simulink model "Symmetry_Inverter"  (Simulink 8.3)
settings: Solver=ode23tb  StartTime=0.0  StopTime=tfin  RelTol=1e-4
values from neighbouring files (symbols this model uses):
  amp_feedback_saturation = 400    [Symmetry_ini_COPY.m]
  Butterworth_filter_order = 8    [Sketch_controller_model_ini.m]    (also in Symmetry_ini.m; Symmetry_ini_COPY.m)
  C_Network = [0, 0, 0]    [Symmetry_ini.m]    (also in Symmetry_ini_COPY.m)
  Capacitive_Load_R_RC = [30e-3,  60e-3,  40e-3;                                1e-3, 5e-3, 3e-3]    [Symmetry_ini.m]    (also in Symmetry_ini_COPY.m = [60e-3,  120e-3,  80e-3;                                 1e-)
  Capacitive_Load_S_RC = [30e-3,  60e-3,  40e-3;                                1e-3, 5e-3, 3e-3]    [Symmetry_ini.m]    (also in Symmetry_ini_COPY.m = [60e-3,  120e-3,  80e-3;                                1e-3)
  Capacitive_Load_T_RC = [30e-3,  60e-3,  40e-3;                                1e-3, 5e-3, 3e-3]    [Symmetry_ini.m]    (also in Symmetry_ini_COPY.m = [60e-3,  120e-3,  80e-3;                                 1e-)
  i = str2num(answer{1})/sample    [Test_intersect.m]
  initial_value = [0.00,0.00,0.00,                  0,0,0]    [Symmetry_ini_COPY.m]
  L_Network = [3.185e-3, 3.185e-3, 3.185e-3, 3.185e-3]    [Symmetry_ini.m]    (also in Symmetry_ini_COPY.m)
  L_Source = [3.185e-3, 3.185e-3, 3.185e-3]    [Sketch_controller_model_ini.m]    (also in Symmetry_ini.m; Symmetry_ini_COPY.m)
  Load_R = [50,50,50]    [Symmetry_ini.m]    (also in Symmetry_ini_COPY.m)
  Load_RL = [35.35,   35.35,   35.35;                  0.1125,  0.1125,  0.1125]    [Symmetry_ini.m]    (also in Symmetry_ini_COPY.m = [35.35,   35.35,   35.35;                   0.1125,  0.1125,)
  Load_Wire_Resistance = [0.1,0.2]    [Symmetry_ini.m]    (also in Symmetry_ini_COPY.m)
  P_gain = 0.00001    (= 1e-05)    [Symmetry_ini_COPY.m]
  phase_feedback_saturation = pi    (= 3.14159265359)    [Symmetry_ini_COPY.m]
  Phase_Source = [0,2/3*pi,4/3*pi]    [Sketch_controller_model_ini.m]    (also in Symmetry_REAL_TIME_ini.m = [0,-2/3*pi,-4/3*pi]; Symmetry_ini.m; Symmetry_ini_COPY.m = [0,-2/3*pi,-4/3*pi])
  PowerGain = 2e-3    (= 0.002)    [Symmetry_ini_COPY.m]
  PowerGain_UpperLimit = 10    [Symmetry_ini_COPY.m]
  R_Network = [0.4, 0.4, 0.4, 0.4]    [Symmetry_ini.m]    (also in Symmetry_ini_COPY.m)
  R_Source = [0.4, 0.4, 0.4]    [Sketch_controller_model_ini.m]    (also in Symmetry_ini.m; Symmetry_ini_COPY.m)
  sample = 10e-5    (= 0.0001)    [Inverter_ini.m]    (also in Sketch_controller_model_ini.m; Symmetry_REAL_TIME_ini.m; Symmetry_ini.m; Symmetry_ini_COPY.m)
  Source_Frequency = [50,50,50]    [Sketch_controller_model_ini.m]    (also in Symmetry_ini.m; Symmetry_ini_COPY.m)
  Start_Control = 1    [Symmetry_ini_COPY.m]
  START_Load_R = [0.001,100,100]    [Symmetry_ini_COPY.m]
  START_Load_RC = [100,100,0.001]    [Symmetry_ini_COPY.m]
  START_Load_RL = [100,0.001,100]    [Symmetry_ini_COPY.m]
  step_size = [5,5,5,                  0.36,0.36,0.36]    [Symmetry_ini_COPY.m]
  test_step = [0.5,0.5,0.5,                  0.02,0.02,0.02]    [Symmetry_ini_COPY.m]
  U_PV_MAX = 600    [Symmetry_ini_COPY.m]
  Urms_Source = [230,230,230]    [Sketch_controller_model_ini.m]    (also in Symmetry_REAL_TIME_ini.m; Symmetry_ini.m; Symmetry_ini_COPY.m)
libraries: powerlib x95, simulink x18, powerlib_extras x12, dspsigops x10, commsequence2 x6, dsparch4 x4, dspxfrm3 x3, powerlib_meascontrol x2
(part 1 of 2)
settings Model: Creator=gorbep  LastModifiedBy=Templomos  SimulationMode=accelerator
settings SolverCC: SolverResetMethod=Robust
settings DataIOCC: SignalLoggingSaveFormat=Dataset
settings OptimizationCC: SimCompilerOptimization=On
settings DebuggingCC: UnderspecifiedInitializationDetection=Simplified  StateNameClashWarn=none
settings GRTTargetCC: CombineOutputUpdateFcns=on  GRTInterface=off

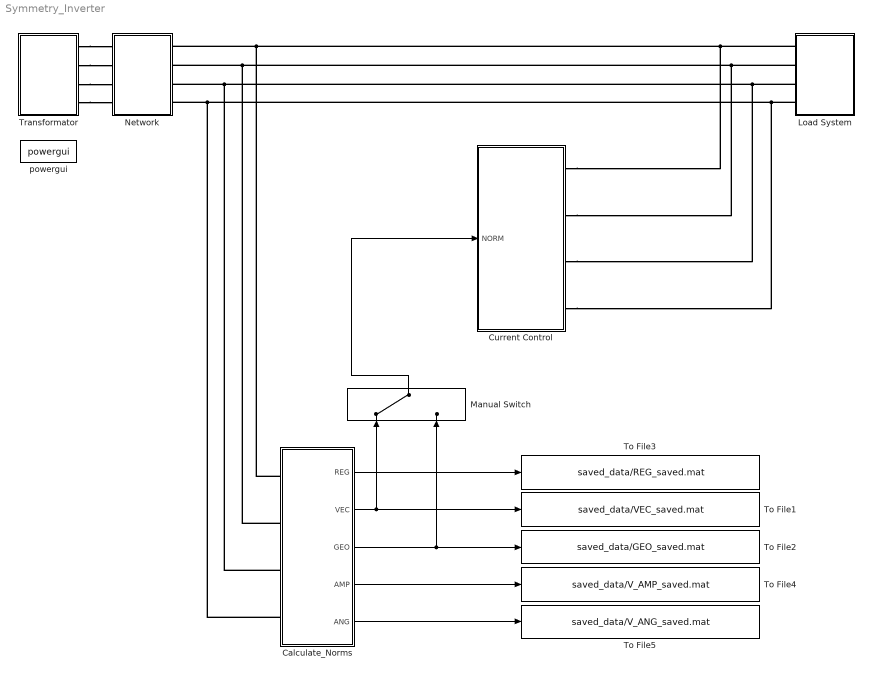
== system Symmetry_Inverter ==
  Calculate_Norms : Subsystem
  Current Control : Subsystem
  Load System : Subsystem
  Manual Switch : ManualSwitch
  Network : Subsystem
  To File1 : ToFile  Filename=saved_data/VEC_saved.mat  MatrixName=VEC_saved  SaveFormat=Timeseries  SampleTime=sample
  To File2 : ToFile  Filename=saved_data/GEO_saved.mat  MatrixName=GEO_saved  SaveFormat=Timeseries  SampleTime=sample
  To File3 : ToFile  Filename=saved_data/REG_saved.mat  MatrixName=REG_saved  SaveFormat=Timeseries  SampleTime=sample
  To File4 : ToFile  Filename=saved_data/V_AMP_saved.mat  MatrixName=V_AMP_saved  SaveFormat=Timeseries  SampleTime=sample
  To File5 : ToFile  Filename=saved_data/V_ANG_saved.mat  MatrixName=V_ANG_saved  SaveFormat=Timeseries  SampleTime=sample
  Transformator : Subsystem
  powergui : powerlib/powergui  SimulationMode=Continuous  SolverType=Tustin  SampleTime=50e-6  frequency=60  SPID=off  DisableSnubberDevices=off  DisableRonSwitches=off  DisableVfSwitches=off  SwTol=0  Interpol=off  DisplayEquations=off  Ts=0  methode=off  frequencyindice=0  Pbase=100e6  ErrMax=1e-4  Iterations=50  UnitsV=kV  UnitsW=MW  FunctionMessages=off  echomessages=off  HookPort=off  EnableUseOfTLC=off  x0status=blocks  RestoreLinks=warning  ResistiveCurrentMeasurement=off  Frange=[0:2:500]  Ylog=off  Xlog=on  ShowGrid=off  save=off  variable=ZData  structure=0  ZoomFFT=on  StartTime=0.0  cycles=1  DisplayStyle=1  fundamental=60  FreqAxis=off  MaxFrequency=1000  frequencyindicesteady=1  RmsSteady=1  display=off
  wires:
  Calculate_Norms/1(REG) -> To File3/1
  Calculate_Norms/3(GEO) -> Manual Switch/2, To File2/1
  Calculate_Norms/2(VEC) -> Manual Switch/1, To File1/1
  Calculate_Norms/4(AMP) -> To File4/1
  Calculate_Norms/5(ANG) -> To File5/1
  Manual Switch/1 -> Current Control/1(NORM)
  connections:
  Transformator/RConn1 -- Network/LConn1
  Transformator/RConn2 -- Network/LConn2
  Transformator/RConn3 -- Network/LConn3
  Transformator/RConn4 -- Network/LConn4
  Load System/LConn1 -- Calculate_Norms/LConn1 -- Network/RConn1 -- Current Control/RConn1
  Load System/LConn2 -- Calculate_Norms/LConn2 -- Network/RConn2 -- Current Control/RConn2
  Load System/LConn3 -- Calculate_Norms/LConn3 -- Network/RConn3 -- Current Control/RConn3
  Load System/LConn4 -- Network/RConn4 -- Calculate_Norms/LConn4 -- Current Control/RConn4

== system Symmetry_Inverter/Calculate_Norms ==
  Mearusement_calc : Subsystem
  Sources1 : ToWorkspace  VariableName=V_conn  SaveFormat=Structure With Time  SampleTime=sample
  Voltage Measurement : powerlib/Measurements/Voltage Measurement  PhasorSimulation=off  OutputType=Complex  PSBequivalent=0
  Voltage Measurement1 : powerlib/Measurements/Voltage Measurement  PhasorSimulation=off  OutputType=Complex  PSBequivalent=0
  Voltage Measurement2 : powerlib/Measurements/Voltage Measurement  PhasorSimulation=off  OutputType=Complex  PSBequivalent=0
  R : PMIOPort  Port=1  Side=Left
  S : PMIOPort  Port=2  Side=Left
  T : PMIOPort  Port=3  Side=Left
  N : PMIOPort  Port=4  Side=Left
  REG : Outport
  VEC : Outport  Port=2
  GEO : Outport  Port=3
  AMP : Outport  Port=4
  ANG : Outport  Port=5
  wires:
  Voltage Measurement/1 -> Mearusement_calc/1(V_R)
  Voltage Measurement1/1 -> Mearusement_calc/2(V_S)
  Voltage Measurement2/1 -> Mearusement_calc/3(V_T)
  Mearusement_calc/1(Voltage) -> Sources1/1
  Mearusement_calc/4(Regular) -> REG/1
  Mearusement_calc/5(Vectorial) -> VEC/1
  Mearusement_calc/6(Geometrial) -> GEO/1
  Mearusement_calc/2(Amplitude) -> AMP/1
  Mearusement_calc/3(Angle) -> ANG/1
  connections:
  Voltage Measurement2/LConn1 -- T/RConn1
  Voltage Measurement2/LConn2 -- Voltage Measurement/LConn2 -- Voltage Measurement1/LConn2 -- N/RConn1
  Voltage Measurement/LConn1 -- R/RConn1
  Voltage Measurement1/LConn1 -- S/RConn1

== system Symmetry_Inverter/Current Control ==
  NORM : Inport
  Abs : Abs
  Current_Sources : Subsystem
  Gain : Gain  Gain=PowerGain
  P(t) Filter3 : dsparch4/Analog Filter Design  method=Butterworth  filttype=Lowpass  N=8  Wlo=200  Whi=80  Rp=2  Rs=40
  Saturation : Saturate  UpperLimit=PowerGain_UpperLimit  LowerLimit=0
  To File4 : ToFile  Filename=saved_data/k_normalised_saved.mat  MatrixName=k_normalised_saved  SaveFormat=Timeseries  SampleTime=sample
  controller : Subsystem
  U : PMIOPort  Port=1  Side=Right
  V : PMIOPort  Port=2  Side=Right
  W : PMIOPort  Port=3  Side=Right
  n : PMIOPort  Port=4  Side=Right
  wires:
  NORM/1 -> controller/2(NORM)
  Gain/1 -> Saturation/1
  Current_Sources/1(k) -> Gain/1
  Saturation/1 -> P(t) Filter3/1
  P(t) Filter3/1 -> Abs/1
  Abs/1 -> controller/1(k), To File4/1
  controller/1(Conteol_Current) -> Current_Sources/1(In1)
  connections:
  n/RConn1 -- Current_Sources/RConn4
  U/RConn1 -- Current_Sources/RConn1
  V/RConn1 -- Current_Sources/RConn2
  W/RConn1 -- Current_Sources/RConn3

== system Symmetry_Inverter/Load System ==
  Conncection_Measurements : Subsystem
  Loads : Subsystem
  Log_Signals : Subsystem
  Wire_resistance_1 : Subsystem
  Wire_resistance_2 : Subsystem
  R : PMIOPort  Port=1  Side=Left
  S : PMIOPort  Port=2  Side=Left
  T : PMIOPort  Port=3  Side=Left
  N : PMIOPort  Port=4  Side=Left
  wires:
  Conncection_Measurements/2(I_abc) -> Log_Signals/2(I_ABC)
  Conncection_Measurements/1(V_abc) -> Log_Signals/1(V_ABC)
  Conncection_Measurements/3(V_line-to-line) -> Log_Signals/3(V_line-to-line)
  connections:
  Conncection_Measurements/RConn1 -- Wire_resistance_2/LConn1
  Conncection_Measurements/RConn2 -- Wire_resistance_2/LConn2
  Conncection_Measurements/RConn3 -- Wire_resistance_2/LConn3
  Wire_resistance_1/LConn1 -- R/RConn1
  Wire_resistance_1/LConn2 -- S/RConn1
  Wire_resistance_1/LConn3 -- T/RConn1
  Wire_resistance_1/LConn4 -- N/RConn1
  Conncection_Measurements/LConn1 -- Wire_resistance_1/RConn1
  Conncection_Measurements/LConn2 -- Wire_resistance_1/RConn2
  Conncection_Measurements/LConn3 -- Wire_resistance_1/RConn3
  Wire_resistance_2/RConn1 -- Loads/LConn1
  Wire_resistance_2/RConn2 -- Loads/LConn2
  Wire_resistance_2/RConn3 -- Loads/LConn3
  Wire_resistance_2/RConn4 -- Loads/LConn4
  Wire_resistance_1/RConn4 -- Conncection_Measurements/LConn4
  Wire_resistance_2/LConn4 -- Conncection_Measurements/RConn4

== system Symmetry_Inverter/Network ==
  Transf-L  Line -R1 : powerlib/Elements/Series RLC Branch  LConnTagsString=__new0  RConnTagsString=__new0  BranchType=RL  Resistance=R_Network(1)  Inductance=L_Network(1)  SetiL0=off  InitialCurrent=0  Capacitance=1.0  Setx0=off  InitialVoltage=0  Measurements=None
  Transf-L  Line -R2 : powerlib/Elements/Series RLC Branch  LConnTagsString=__new0  RConnTagsString=__new0  BranchType=RL  Resistance=R_Network(2)  Inductance=L_Network(2)  SetiL0=off  InitialCurrent=0  Capacitance=1.0  Setx0=off  InitialVoltage=0  Measurements=None
  Transf-L  Line -R3 : powerlib/Elements/Series RLC Branch  LConnTagsString=__new0  RConnTagsString=__new0  BranchType=RL  Resistance=R_Network(3)  Inductance=L_Network(3)  SetiL0=off  InitialCurrent=0  Capacitance=1.0  Setx0=off  InitialVoltage=0  Measurements=None
  Transf-L  Line -R4 : powerlib/Elements/Series RLC Branch  LConnTagsString=__new0  RConnTagsString=__new0  BranchType=C  Resistance=i  Inductance=0.003185  SetiL0=off  InitialCurrent=0  Capacitance=C_Network(1)  Setx0=off  InitialVoltage=0  Measurements=None
  Transf-L  Line -R5 : powerlib/Elements/Series RLC Branch  LConnTagsString=__new0  RConnTagsString=__new0  BranchType=C  Resistance=i  Inductance=0.003185  SetiL0=off  InitialCurrent=0  Capacitance=C_Network(2)  Setx0=off  InitialVoltage=0  Measurements=None
  Transf-L  Line -R7 : powerlib/Elements/Series RLC Branch  LConnTagsString=__new0  RConnTagsString=__new0  BranchType=C  Resistance=i  Inductance=0.003185  SetiL0=off  InitialCurrent=0  Capacitance=C_Network(2)  Setx0=off  InitialVoltage=0  Measurements=None
  Transf-L  Line -R9 : powerlib/Elements/Series RLC Branch  LConnTagsString=__new0  RConnTagsString=__new0  BranchType=RL  Resistance=R_Network(4)  Inductance=L_Network(4)  SetiL0=off  InitialCurrent=0  Capacitance=1.0  Setx0=off  InitialVoltage=0  Measurements=None
  R : PMIOPort  Port=1  Side=Left
  U : PMIOPort  Port=2  Side=Right
  S : PMIOPort  Port=3  Side=Left
  V : PMIOPort  Port=4  Side=Right
  T : PMIOPort  Port=5  Side=Left
  W : PMIOPort  Port=6  Side=Right
  N : PMIOPort  Port=7  Side=Left
  n : PMIOPort  Port=8  Side=Right
  connections:
  Transf-L  Line -R4/LConn1 -- U/RConn1 -- Transf-L  Line -R1/RConn1
  Transf-L  Line -R2/RConn1 -- V/RConn1 -- Transf-L  Line -R5/LConn1
  Transf-L  Line -R7/LConn1 -- W/RConn1 -- Transf-L  Line -R3/RConn1
  Transf-L  Line -R3/LConn1 -- T/RConn1
  Transf-L  Line -R2/LConn1 -- S/RConn1
  R/RConn1 -- Transf-L  Line -R1/LConn1
  n/RConn1 -- Transf-L  Line -R4/RConn1 -- Transf-L  Line -R5/RConn1 -- Transf-L  Line -R7/RConn1 -- Transf-L  Line -R9/RConn1
  Transf-L  Line -R9/LConn1 -- N/RConn1

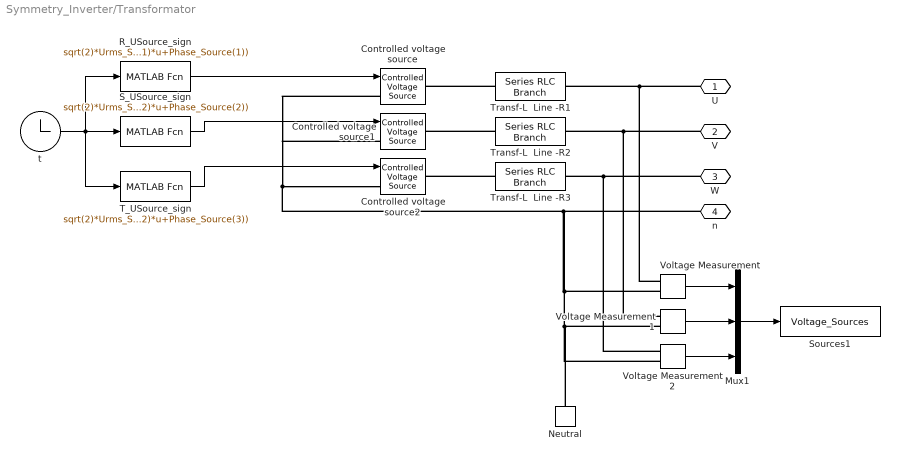
== system Symmetry_Inverter/Transformator ==
  " R_USource_sign" : MATLABFcn  MATLABFcn=sqrt(2)*Urms_Source(1)*sin(2*pi*Source_Frequency(1)*u+Phase_Source(1))  SampleTime=sample
  " S_USource_sign" : MATLABFcn  MATLABFcn=sqrt(2)*Urms_Source(2)*sin(2*pi*Source_Frequency(2)*u+Phase_Source(2))  SampleTime=sample
  " T_USource_sign" : MATLABFcn  MATLABFcn=sqrt(2)*Urms_Source(3)*sin(2*pi*Source_Frequency(2)*u+Phase_Source(3))  SampleTime=sample
  Controlled voltage source : powerlib/Electrical Sources/Controlled Voltage Source  Initialize=off  Source_Type=AC  Amplitude=0  Phase=0  Frequency=0  Measurements=None
  Controlled voltage source1 : powerlib/Electrical Sources/Controlled Voltage Source  Initialize=off  Source_Type=AC  Amplitude=0  Phase=0  Frequency=0  Measurements=None
  Controlled voltage source2 : powerlib/Electrical Sources/Controlled Voltage Source  Initialize=off  Source_Type=AC  Amplitude=0  Phase=0  Frequency=0  Measurements=None
  Mux1 : Mux  Inputs=3
  Neutral : powerlib/Elements/Neutral  LConnTagsString=a  NodeNumber=10
  Sources1 : ToWorkspace  VariableName=Voltage_Sources  SaveFormat=Structure With Time  SampleTime=-1
  Transf-L  Line -R1 : powerlib/Elements/Series RLC Branch  LConnTagsString=__new0  RConnTagsString=__new0  BranchType=RL  Resistance=R_Source(1)  Inductance=L_Source(1)  SetiL0=off  InitialCurrent=0  Capacitance=1.0  Setx0=off  InitialVoltage=0  Measurements=None
  Transf-L  Line -R2 : powerlib/Elements/Series RLC Branch  LConnTagsString=__new0  RConnTagsString=__new0  BranchType=RL  Resistance=R_Source(2)  Inductance=L_Source(2)  SetiL0=off  InitialCurrent=0  Capacitance=1.0  Setx0=off  InitialVoltage=0  Measurements=None
  Transf-L  Line -R3 : powerlib/Elements/Series RLC Branch  LConnTagsString=__new0  RConnTagsString=__new0  BranchType=RL  Resistance=R_Source(3)  Inductance=L_Source(3)  SetiL0=off  InitialCurrent=0  Capacitance=1.0  Setx0=off  InitialVoltage=0  Measurements=None
  Voltage Measurement : powerlib/Measurements/Voltage Measurement  PhasorSimulation=off  OutputType=Complex  PSBequivalent=0
  Voltage Measurement1 : powerlib/Measurements/Voltage Measurement  PhasorSimulation=off  OutputType=Complex  PSBequivalent=0
  Voltage Measurement2 : powerlib/Measurements/Voltage Measurement  PhasorSimulation=off  OutputType=Complex  PSBequivalent=0
  t : Clock
      settings: Decimation=CLK
  U : PMIOPort  Port=1  Side=Right
  V : PMIOPort  Port=2  Side=Right
  W : PMIOPort  Port=3  Side=Right
  n : PMIOPort  Port=4  Side=Right
  wires:
  " R_USource_sign"/1 -> Controlled voltage source/1
  " S_USource_sign"/1 -> Controlled voltage source1/1
  " T_USource_sign"/1 -> Controlled voltage source2/1
  t/1 -> " R_USource_sign"/1, " T_USource_sign"/1, " S_USource_sign"/1
  Voltage Measurement/1 -> Mux1/1
  Voltage Measurement1/1 -> Mux1/2
  Voltage Measurement2/1 -> Mux1/3
  Mux1/1 -> Sources1/1
  connections:
  n/RConn1 -- Neutral/LConn1 -- Voltage Measurement2/LConn2 -- Voltage Measurement1/LConn2 -- Voltage Measurement/LConn2 -- Controlled voltage source/LConn1 -- Controlled voltage source1/LConn1 -- Controlled voltage source2/LConn1
  Transf-L  Line -R2/LConn1 -- Controlled voltage source1/RConn1
  Transf-L  Line -R3/LConn1 -- Controlled voltage source2/RConn1
  Transf-L  Line -R1/LConn1 -- Controlled voltage source/RConn1
  U/RConn1 -- Voltage Measurement/LConn1 -- Transf-L  Line -R1/RConn1
  V/RConn1 -- Voltage Measurement1/LConn1 -- Transf-L  Line -R2/RConn1
  W/RConn1 -- Voltage Measurement2/LConn1 -- Transf-L  Line -R3/RConn1

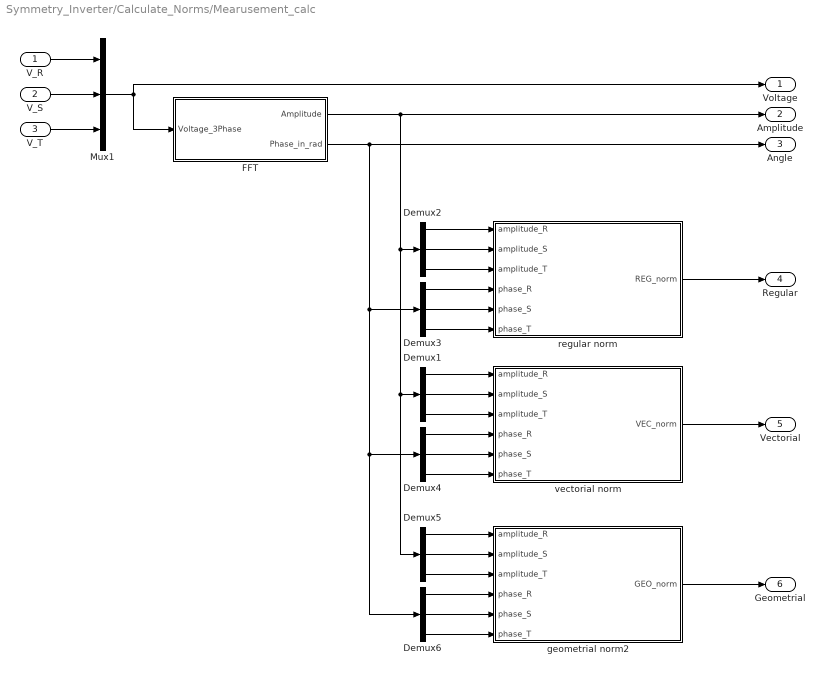
== system Symmetry_Inverter/Calculate_Norms/Mearusement_calc ==
  V_R : Inport
  V_S : Inport  Port=2
  V_T : Inport  Port=3
  Demux{1..6} (6 alike) : Demux  Outputs=3
  FFT : Subsystem
  Mux1 : Mux  Inputs=3
  geometrial norm2 : MATLAB Function  TreatAsAtomicUnit=on
  regular norm : MATLAB Function  TreatAsAtomicUnit=on
  vectorial norm : MATLAB Function  TreatAsAtomicUnit=on
  Voltage : Outport
  Amplitude : Outport  Port=2
  Angle : Outport  Port=3
  Regular : Outport  Port=4
  Vectorial : Outport  Port=5
  Geometrial : Outport  Port=6
  wires:
  V_R/1 -> Mux1/1
  V_T/1 -> Mux1/3
  Mux1/1 -> Voltage/1, FFT/1(Voltage_3Phase)
  V_S/1 -> Mux1/2
  regular norm/1(REG_norm) -> Regular/1
  Demux2/1 -> regular norm/1(amplitude_R)
  Demux2/2 -> regular norm/2(amplitude_S)
  Demux2/3 -> regular norm/3(amplitude_T)
  Demux3/1 -> regular norm/4(phase_R)
  Demux3/2 -> regular norm/5(phase_S)
  Demux3/3 -> regular norm/6(phase_T)
  Demux1/1 -> vectorial norm/1(amplitude_R)
  Demux1/2 -> vectorial norm/2(amplitude_S)
  Demux1/3 -> vectorial norm/3(amplitude_T)
  Demux4/1 -> vectorial norm/4(phase_R)
  Demux4/2 -> vectorial norm/5(phase_S)
  Demux4/3 -> vectorial norm/6(phase_T)
  vectorial norm/1(VEC_norm) -> Vectorial/1
  FFT/1(Amplitude) -> Amplitude/1, Demux5/1, Demux1/1, Demux2/1
  FFT/2(Phase_in_rad) -> Angle/1, Demux6/1, Demux4/1, Demux3/1
  Demux5/1 -> geometrial norm2/1(amplitude_R)
  Demux5/2 -> geometrial norm2/2(amplitude_S)
  Demux5/3 -> geometrial norm2/3(amplitude_T)
  Demux6/1 -> geometrial norm2/4(phase_R)
  Demux6/2 -> geometrial norm2/5(phase_S)
  Demux6/3 -> geometrial norm2/6(phase_T)
  geometrial norm2/1(GEO_norm) -> Geometrial/1

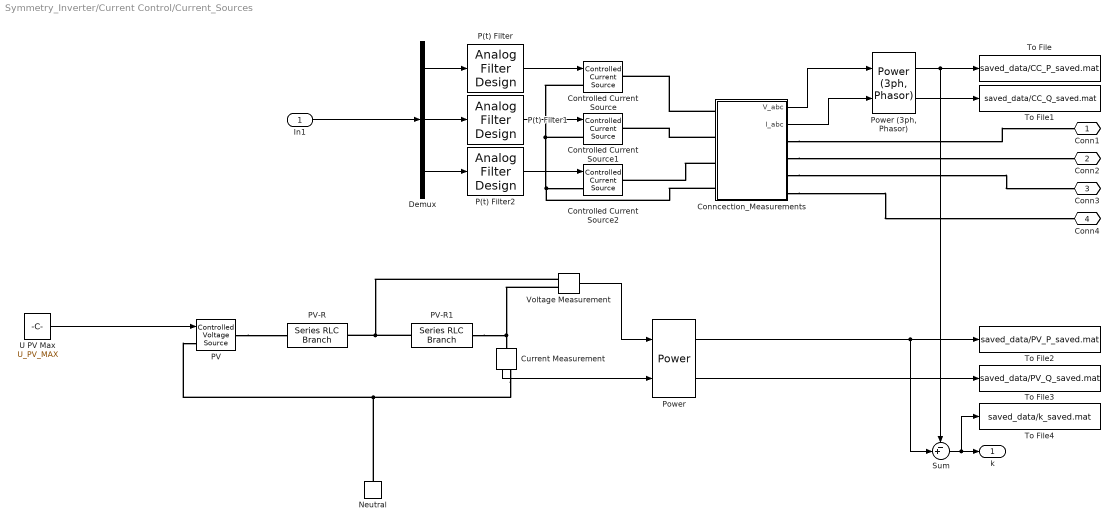
== system Symmetry_Inverter/Current Control/Current_Sources ==
  In1 : Inport
  Conncection_Measurements : Subsystem
  Controlled Current Source : powerlib/Electrical Sources/Controlled Current Source  Initialize=on  Source_Type=AC  Amplitude=0  Phase=0  Frequency=0  Measurements=None
  Controlled Current Source1 : powerlib/Electrical Sources/Controlled Current Source  Initialize=on  Source_Type=AC  Amplitude=0  Phase=0  Frequency=0  Measurements=None
  Controlled Current Source2 : powerlib/Electrical Sources/Controlled Current Source  Initialize=on  Source_Type=AC  Amplitude=0  Phase=0  Frequency=0  Measurements=None
  Current Measurement : powerlib/Measurements/Current Measurement  PhasorSimulation=off  OutputType=Complex  PSBequivalent=0
  Demux : Demux  Outputs=3
  Neutral : powerlib/Elements/Neutral  LConnTagsString=a  NodeNumber=10
  P(t) Filter : dsparch4/Analog Filter Design  method=Butterworth  filttype=Lowpass  N=Butterworth_filter_order  Wlo=Butterworth_passband_frequency  Whi=80  Rp=2  Rs=40
  P(t) Filter1 : dsparch4/Analog Filter Design  method=Butterworth  filttype=Lowpass  N=Butterworth_filter_order  Wlo=Butterworth_passband_frequency  Whi=80  Rp=2  Rs=40
  P(t) Filter2 : dsparch4/Analog Filter Design  method=Butterworth  filttype=Lowpass  N=Butterworth_filter_order  Wlo=Butterworth_passband_frequency  Whi=80  Rp=2  Rs=40
  PV : powerlib/Electrical Sources/Controlled Voltage Source  Initialize=off  Source_Type=AC  Amplitude=0  Phase=0  Frequency=0  Measurements=None
  PV-R : powerlib/Elements/Series RLC Branch  LConnTagsString=__new0  RConnTagsString=__new0  BranchType=R  Resistance=5  Inductance=0.1  SetiL0=off  InitialCurrent=0  Capacitance=1.0  Setx0=off  InitialVoltage=0  Measurements=None
  PV-R1 : powerlib/Elements/Series RLC Branch  LConnTagsString=__new0  RConnTagsString=__new0  BranchType=R  Resistance=5  Inductance=0.1  SetiL0=off  InitialCurrent=0  Capacitance=1.0  Setx0=off  InitialVoltage=0  Measurements=None
  Power : powerlib_meascontrol/Measurements/Power  Freq=60  Vinit=[1, 0]  Iinit=[1, 0]  Ts=0
  "Power (3ph, Phasor)" : powerlib_meascontrol/Measurements/Power (3ph, Phasor)
  Sum : Sum  Inputs=-+|
  To File : ToFile  Filename=saved_data/CC_P_saved.mat  MatrixName=CC_P_saved  SaveFormat=Timeseries  SampleTime=sample
  To File1 : ToFile  Filename=saved_data/CC_Q_saved.mat  MatrixName=CC_Q_saved  SaveFormat=Timeseries  SampleTime=sample
  To File2 : ToFile  Filename=saved_data/PV_P_saved.mat  MatrixName=PV_P_saved  SaveFormat=Timeseries  SampleTime=sample
  To File3 : ToFile  Filename=saved_data/PV_Q_saved.mat  MatrixName=PV_Q_saved  SaveFormat=Timeseries  SampleTime=sample
  To File4 : ToFile  Filename=saved_data/k_saved.mat  MatrixName=k_saved  SaveFormat=Timeseries  SampleTime=sample
  U PV Max : Constant  Value=U_PV_MAX
  Voltage Measurement : powerlib/Measurements/Voltage Measurement  PhasorSimulation=off  OutputType=Complex  PSBequivalent=0
  Conn1 : PMIOPort  Port=1  Side=Right
  Conn2 : PMIOPort  Port=2  Side=Right
  Conn3 : PMIOPort  Port=3  Side=Right
  Conn4 : PMIOPort  Port=4  Side=Right
  k : Outport
  wires:
  In1/1 -> Demux/1
  Demux/1 -> P(t) Filter/1
  Demux/2 -> P(t) Filter1/1
  Demux/3 -> P(t) Filter2/1
  P(t) Filter/1 -> Controlled Current Source/1
  P(t) Filter1/1 -> Controlled Current Source1/1
  P(t) Filter2/1 -> Controlled Current Source2/1
  Voltage Measurement/1 -> Power/1
  "Power (3ph, Phasor)"/2 -> To File1/1
  Power/1 -> Sum/2, To File2/1
  Power/2 -> To File3/1
  U PV Max/1 -> PV/1
  Current Measurement/1 -> Power/2
  Conncection_Measurements/2(I_abc) -> "Power (3ph, Phasor)"/2
  Conncection_Measurements/1(V_abc) -> "Power (3ph, Phasor)"/1
  Sum/1 -> k/1, To File4/1
  "Power (3ph, Phasor)"/1 -> Sum/1, To File/1
  connections:
  Controlled Current Source/LConn1 -- Controlled Current Source1/LConn1 -- Conncection_Measurements/LConn4 -- Controlled Current Source2/LConn1
  PV/RConn1 -- PV-R/LConn1
  PV-R1/LConn1 -- Voltage Measurement/LConn1 -- PV-R/RConn1
  Current Measurement/RConn1 -- Neutral/LConn1 -- PV/LConn1
  Conncection_Measurements/LConn1 -- Controlled Current Source/RConn1
  Conncection_Measurements/LConn2 -- Controlled Current Source1/RConn1
  Conncection_Measurements/LConn3 -- Controlled Current Source2/RConn1
  Conncection_Measurements/RConn4 -- Conn4/RConn1
  Conncection_Measurements/RConn3 -- Conn3/RConn1
  Conncection_Measurements/RConn2 -- Conn2/RConn1
  Conncection_Measurements/RConn1 -- Conn1/RConn1
  PV-R1/RConn1 -- Voltage Measurement/LConn2 -- Current Measurement/LConn1

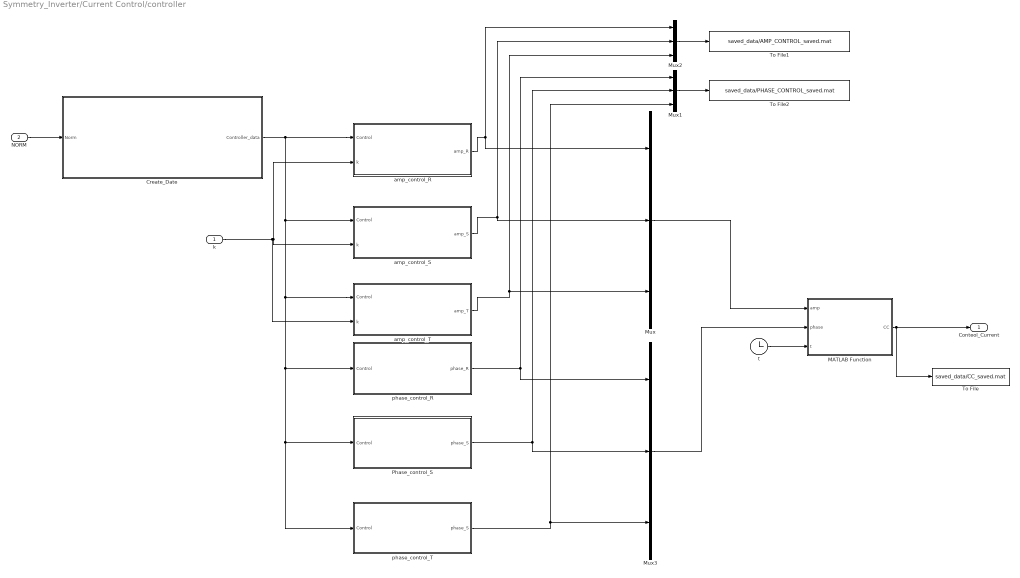
== system Symmetry_Inverter/Current Control/controller ==
  k : Inport
  NORM : Inport  Port=2
  Create_Date : Subsystem
  MATLAB Function : MATLAB Function  TreatAsAtomicUnit=on
  Mux{,1..3} (4 alike) : Mux  Inputs=3
  Phase_control_S : Subsystem
  To File : ToFile  Filename=saved_data/CC_saved.mat  MatrixName=CC_saved  SaveFormat=Timeseries  SampleTime=sample
  To File1 : ToFile  Filename=saved_data/AMP_CONTROL_saved.mat  MatrixName=AMP_CONTROL_saved  SaveFormat=Timeseries  SampleTime=sample
  To File2 : ToFile  Filename=saved_data/PHASE_CONTROL_saved.mat  MatrixName=PHASE_CONTROL_saved  SaveFormat=Timeseries  SampleTime=sample
  amp_control_R : Subsystem
  amp_control_S : Subsystem
  amp_control_T : Subsystem
  phase_control_R : Subsystem
  phase_control_T : Subsystem
  t : Clock
      settings: Decimation=CLK
  Conteol_Current : Outport
  wires:
  amp_control_S/1(amp_S) -> Mux/2, Mux2/2
  amp_control_T/1(amp_T) -> Mux2/3, Mux/3
  Create_Date/1(Controller_data) -> phase_control_T/1(Control), Phase_control_S/1(Control), phase_control_R/1(Control), amp_control_T/1(Control), amp_control_S/1(Control), amp_control_R/1(Control)
  amp_control_R/1(amp_R) -> Mux/1, Mux2/1
  Phase_control_S/1(phase_S) -> Mux3/2, Mux1/2
  phase_control_T/1(phase_S) -> Mux3/3, Mux1/3
  Mux1/1 -> To File2/1
  phase_control_R/1(phase_R) -> Mux3/1, Mux1/1
  Mux2/1 -> To File1/1
  NORM/1 -> Create_Date/1(Norm)
  t/1 -> MATLAB Function/3(t)
  MATLAB Function/1(CC) -> Conteol_Current/1, To File/1
  Mux/1 -> MATLAB Function/1(amp)
  Mux3/1 -> MATLAB Function/2(phase)
  k/1 -> amp_control_T/2(k), amp_control_R/2(k), amp_control_S/2(k)

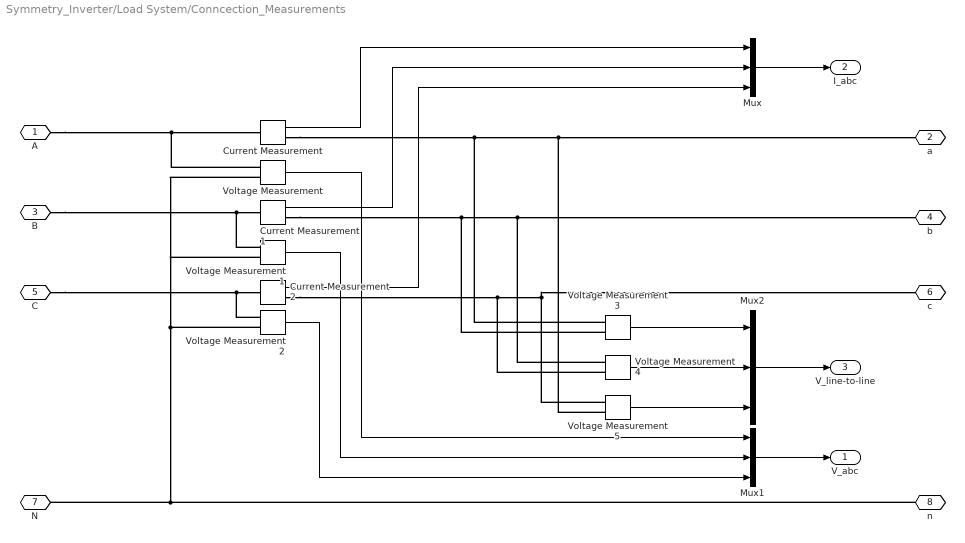
== system Symmetry_Inverter/Load System/Conncection_Measurements ==
  Current Measurement : powerlib/Measurements/Current Measurement  PhasorSimulation=off  OutputType=Complex  PSBequivalent=0
  Current Measurement1 : powerlib/Measurements/Current Measurement  PhasorSimulation=off  OutputType=Complex  PSBequivalent=0
  Current Measurement2 : powerlib/Measurements/Current Measurement  PhasorSimulation=off  OutputType=Complex  PSBequivalent=0
  Mux : Mux  Inputs=3
  Mux1 : Mux  Inputs=3
  Mux2 : Mux  Inputs=3
  Voltage Measurement{,1..5} (6 alike) : powerlib/Measurements/Voltage Measurement  PhasorSimulation=off  OutputType=Complex  PSBequivalent=0
  A : PMIOPort  Port=1  Side=Left
  a : PMIOPort  Port=2  Side=Right
  B : PMIOPort  Port=3  Side=Left
  b : PMIOPort  Port=4  Side=Right
  C : PMIOPort  Port=5  Side=Left
  c : PMIOPort  Port=6  Side=Right
  N : PMIOPort  Port=7  Side=Left
  n : PMIOPort  Port=8  Side=Right
  V_abc : Outport
  I_abc : Outport  Port=2
  V_line-to-line : Outport  Port=3
  wires:
  Current Measurement1/1 -> Mux/2
  Mux1/1 -> V_abc/1
  Mux/1 -> I_abc/1
  Current Measurement/1 -> Mux/1
  Voltage Measurement/1 -> Mux1/1
  Current Measurement2/1 -> Mux/3
  Voltage Measurement1/1 -> Mux1/2
  Voltage Measurement2/1 -> Mux1/3
  Mux2/1 -> V_line-to-line/1
  Voltage Measurement3/1 -> Mux2/1
  Voltage Measurement4/1 -> Mux2/2
  Voltage Measurement5/1 -> Mux2/3
  connections:
  Current Measurement2/RConn1 -- Voltage Measurement5/LConn1 -- c/RConn1 -- Voltage Measurement4/LConn2
  Current Measurement/RConn1 -- Voltage Measurement5/LConn2 -- a/RConn1 -- Voltage Measurement3/LConn1
  Current Measurement1/RConn1 -- Voltage Measurement3/LConn2 -- Voltage Measurement4/LConn1 -- b/RConn1
  Voltage Measurement2/LConn1 -- C/RConn1 -- Current Measurement2/LConn1
  Voltage Measurement2/LConn2 -- Voltage Measurement1/LConn2 -- Voltage Measurement/LConn2 -- N/RConn1 -- n/RConn1
  Voltage Measurement1/LConn1 -- B/RConn1 -- Current Measurement1/LConn1
  Voltage Measurement/LConn1 -- A/RConn1 -- Current Measurement/LConn1

== system Symmetry_Inverter/Load System/Loads ==
  Capacitive_Loads_RST : Subsystem
  Inductive_Loads_RST : Subsystem
  Ohmic_Loads_RST : Subsystem
  R : PMIOPort  Port=1  Side=Left
  S : PMIOPort  Port=2  Side=Left
  T : PMIOPort  Port=3  Side=Left
  N : PMIOPort  Port=4  Side=Left
  connections:
  Ohmic_Loads_RST/LConn1 -- R/RConn1 -- Inductive_Loads_RST/LConn1 -- Capacitive_Loads_RST/RConn1
  Capacitive_Loads_RST/RConn2 -- S/RConn1 -- Inductive_Loads_RST/LConn2 -- Ohmic_Loads_RST/LConn2
  Capacitive_Loads_RST/RConn3 -- T/RConn1 -- Inductive_Loads_RST/LConn3 -- Ohmic_Loads_RST/LConn3
  N/RConn1 -- Inductive_Loads_RST/RConn1 -- Ohmic_Loads_RST/RConn1 -- Capacitive_Loads_RST/LConn1

== system Symmetry_Inverter/Load System/Log_Signals ==
  V_ABC : Inport
  I_ABC : Inport  Port=2
  V_line-to-line : Inport  Port=3
  3_Phase_P_Q : Subsystem
  3_Phase_RMS : Subsystem
  3_Phase_RMS1 : Subsystem
  3_Phase_THD : Subsystem
  To File1 : ToFile  Filename=saved_data/Vrms_saved.mat  MatrixName=Vrms_saved  SaveFormat=Timeseries  SampleTime=sample
  To File2 : ToFile  Filename=saved_data/THD_saved.mat  MatrixName=THD_saved  SaveFormat=Timeseries  SampleTime=sample
  To File3 : ToFile  Filename=saved_data/V_saved.mat  MatrixName=V_saved  SaveFormat=Timeseries  SampleTime=sample
  To File4 : ToFile  Filename=saved_data/PQ_R_saved.mat  MatrixName=PQ_R_saved  SaveFormat=Timeseries  SampleTime=sample
  To File5 : ToFile  Filename=saved_data/Irms_saved.mat  MatrixName=REG_saved  SaveFormat=Timeseries  SampleTime=sample
  To File6 : ToFile  Filename=saved_data/I_saved.mat  MatrixName=I_saved  SaveFormat=Timeseries  SampleTime=sample
  To File7 : ToFile  Filename=saved_data/V_line_saved.mat  MatrixName=V_line_saved  SaveFormat=Timeseries  SampleTime=sample
  To File8 : ToFile  Filename=saved_data/PQ_S_saved.mat  MatrixName=PQ_S_saved  SaveFormat=Timeseries  SampleTime=sample
  To File9 : ToFile  Filename=saved_data/PQ_T_saved.mat  MatrixName=PQ_T_saved  SaveFormat=Timeseries  SampleTime=sample
  wires:
  I_ABC/1 -> To File6/1, 3_Phase_RMS1/1(I_RST), 3_Phase_P_Q/2(I_RMS)
  V_ABC/1 -> To File3/1, 3_Phase_P_Q/1(U_RMS), 3_Phase_RMS/1(U_RST), 3_Phase_THD/1(U_RST)
  3_Phase_RMS1/1(I_RMS) -> To File5/1
  3_Phase_RMS/1(U_RMS) -> To File1/1
  3_Phase_THD/1(THD_RST) -> To File2/1
  V_line-to-line/1 -> To File7/1
  3_Phase_P_Q/1(PQ_R) -> To File4/1
  3_Phase_P_Q/3(PQ_T) -> To File9/1
  3_Phase_P_Q/2(PQ_S) -> To File8/1

== system Symmetry_Inverter/Load System/Wire_resistance_1 ==
  Series RLC Branch{,5..7} (4 alike) : powerlib/Elements/Series RLC Branch  LConnTagsString=__new0  RConnTagsString=__new0  BranchType=R  Resistance=Load_Wire_Resistance(1)  Inductance=1e-3  SetiL0=off  InitialCurrent=0  Capacitance=1e-6  Setx0=off  InitialVoltage=0  Measurements=None
  A : PMIOPort  Port=1  Side=Left
  a : PMIOPort  Port=2  Side=Right
  B : PMIOPort  Port=3  Side=Left
  b : PMIOPort  Port=4  Side=Right
  C : PMIOPort  Port=5  Side=Left
  c : PMIOPort  Port=6  Side=Right
  N : PMIOPort  Port=7  Side=Left
  n : PMIOPort  Port=8  Side=Right
  connections:
  Series RLC Branch7/RConn1 -- n/RConn1
  Series RLC Branch5/LConn1 -- B/RConn1
  Series RLC Branch6/LConn1 -- C/RConn1
  Series RLC Branch/RConn1 -- a/RConn1
  Series RLC Branch/LConn1 -- A/RConn1
  Series RLC Branch7/LConn1 -- N/RConn1
  Series RLC Branch6/RConn1 -- c/RConn1
  Series RLC Branch5/RConn1 -- b/RConn1

== system Symmetry_Inverter/Load System/Wire_resistance_2 ==
  Series RLC Branch{1..4} (4 alike) : powerlib/Elements/Series RLC Branch  LConnTagsString=__new0  RConnTagsString=__new0  BranchType=R  Resistance=Load_Wire_Resistance(2)  Inductance=1e-3  SetiL0=off  InitialCurrent=0  Capacitance=1e-6  Setx0=off  InitialVoltage=0  Measurements=None
  A : PMIOPort  Port=1  Side=Left
  a : PMIOPort  Port=2  Side=Right
  B : PMIOPort  Port=3  Side=Left
  b : PMIOPort  Port=4  Side=Right
  C : PMIOPort  Port=5  Side=Left
  c : PMIOPort  Port=6  Side=Right
  N : PMIOPort  Port=7  Side=Left
  n : PMIOPort  Port=8  Side=Right
  connections:
  Series RLC Branch2/RConn1 -- b/RConn1
  Series RLC Branch1/RConn1 -- a/RConn1
  Series RLC Branch4/RConn1 -- n/RConn1
  Series RLC Branch2/LConn1 -- B/RConn1
  Series RLC Branch3/RConn1 -- c/RConn1
  Series RLC Branch3/LConn1 -- C/RConn1
  Series RLC Branch1/LConn1 -- A/RConn1
  Series RLC Branch4/LConn1 -- N/RConn1

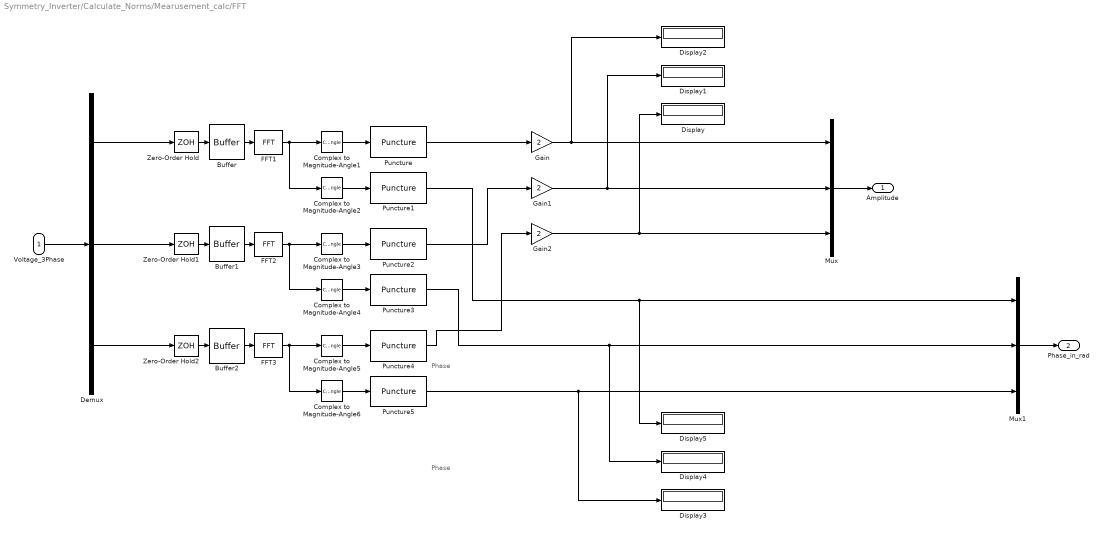
== system Symmetry_Inverter/Calculate_Norms/Mearusement_calc/FFT ==
  note: Phase
  note: Phase
  Voltage_3Phase : Inport
  Buffer : Buffer  N=128  TreatMby1Signals=One channel
  Buffer1 : Buffer  N=128  TreatMby1Signals=One channel
  Buffer2 : Buffer  N=128  TreatMby1Signals=One channel
  Complex to Magnitude-Angle1 : ComplexToMagnitudeAngle  Output=Magnitude
  Complex to Magnitude-Angle2 : ComplexToMagnitudeAngle  Output=Angle
  Complex to Magnitude-Angle3 : ComplexToMagnitudeAngle  Output=Magnitude
  Complex to Magnitude-Angle4 : ComplexToMagnitudeAngle  Output=Angle
  Complex to Magnitude-Angle5 : ComplexToMagnitudeAngle  Output=Magnitude
  Complex to Magnitude-Angle6 : ComplexToMagnitudeAngle  Output=Angle
  Demux : Demux  Outputs=3
  Display{,1..5} (6 alike) : Display
  FFT1 : dspxfrm3/FFT  CompMethod=Table lookup  TableOpt=NEW  TableOptActive=Speed  BitRevOrder=off  InheritFFTLength=on  FFTLength=64  WrapInput=on  RowConvenienceOn=on  FFTImplementation=Auto  SkipNorm=on  firstCoeffDataTypeStr=Inherit: Same word length as input  firstCoeffLastDataTypeStr=Inherit: Same word length as input  outputMin=[]  outputMax=[]  roundingMode=Floor  overflowMode=off
  FFT2 : dspxfrm3/FFT  CompMethod=Table lookup  TableOpt=NEW  TableOptActive=Speed  BitRevOrder=off  InheritFFTLength=on  FFTLength=64  WrapInput=on  RowConvenienceOn=on  FFTImplementation=Auto  SkipNorm=on  firstCoeffDataTypeStr=Inherit: Same word length as input  firstCoeffLastDataTypeStr=Inherit: Same word length as input  outputMin=[]  outputMax=[]  roundingMode=Floor  overflowMode=off
  FFT3 : dspxfrm3/FFT  CompMethod=Table lookup  TableOpt=NEW  TableOptActive=Speed  BitRevOrder=off  InheritFFTLength=on  FFTLength=64  WrapInput=on  RowConvenienceOn=on  FFTImplementation=Auto  SkipNorm=on  firstCoeffDataTypeStr=Inherit: Same word length as input  firstCoeffLastDataTypeStr=Inherit: Same word length as input  outputMin=[]  outputMax=[]  roundingMode=Floor  overflowMode=off
  Gain : Gain  Gain=2  SampleTime=sample
  Gain1 : Gain  Gain=2  SampleTime=sample
  Gain2 : Gain  Gain=2  SampleTime=sample
  Mux : Mux  Inputs=3
  Mux1 : Mux  Inputs=3
  Puncture{,1..5} (6 alike) : commsequence2/Puncture  punctureVector=s'
  Zero-Order Hold : ZeroOrderHold  SampleTime=20e-3/128
  Zero-Order Hold1 : ZeroOrderHold  SampleTime=20e-3/128
  Zero-Order Hold2 : ZeroOrderHold  SampleTime=20e-3/128
  Amplitude : Outport
  Phase_in_rad : Outport  Port=2
  wires:
  FFT1/1 -> Complex to Magnitude-Angle1/1, Complex to Magnitude-Angle2/1
  Buffer/1 -> FFT1/1
  Zero-Order Hold/1 -> Buffer/1
  Complex to Magnitude-Angle1/1 -> Puncture/1
  Complex to Magnitude-Angle2/1 -> Puncture1/1
  FFT2/1 -> Complex to Magnitude-Angle4/1, Complex to Magnitude-Angle3/1
  Buffer1/1 -> FFT2/1
  Zero-Order Hold1/1 -> Buffer1/1
  Complex to Magnitude-Angle3/1 -> Puncture2/1
  Complex to Magnitude-Angle4/1 -> Puncture3/1
  FFT3/1 -> Complex to Magnitude-Angle5/1, Complex to Magnitude-Angle6/1
  Buffer2/1 -> FFT3/1
  Zero-Order Hold2/1 -> Buffer2/1
  Complex to Magnitude-Angle5/1 -> Puncture4/1
  Complex to Magnitude-Angle6/1 -> Puncture5/1
  Voltage_3Phase/1 -> Demux/1
  Demux/2 -> Zero-Order Hold1/1
  Demux/3 -> Zero-Order Hold2/1
  Puncture/1 -> Gain/1
  Puncture2/1 -> Gain1/1
  Puncture4/1 -> Gain2/1
  Puncture1/1 -> Display5/1, Mux1/1
  Puncture3/1 -> Display4/1, Mux1/2
  Puncture5/1 -> Display3/1, Mux1/3
  Mux/1 -> Amplitude/1
  Mux1/1 -> Phase_in_rad/1
  Gain/1 -> Display2/1, Mux/1
  Gain1/1 -> Display1/1, Mux/2
  Gain2/1 -> Display/1, Mux/3
  Demux/1 -> Zero-Order Hold/1

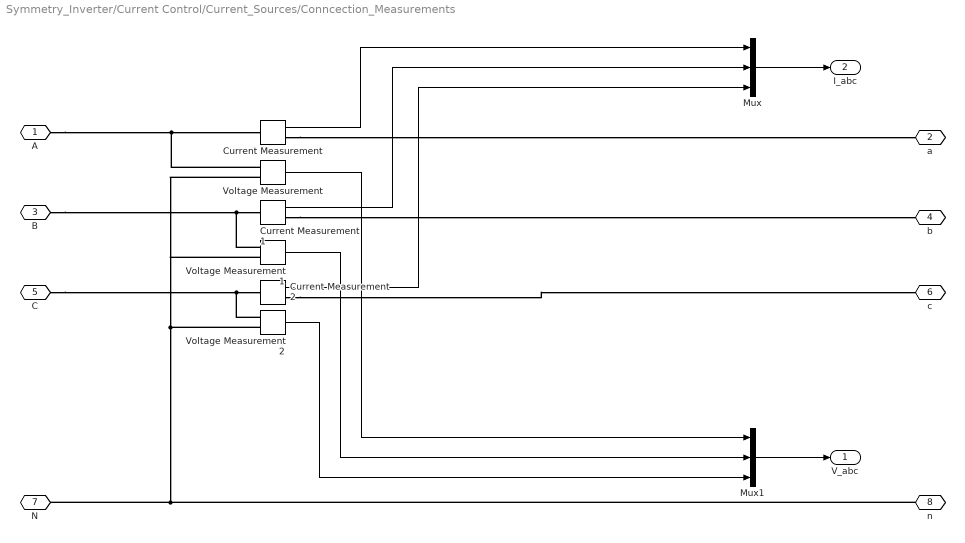
== system Symmetry_Inverter/Current Control/Current_Sources/Conncection_Measurements ==
  Current Measurement : powerlib/Measurements/Current Measurement  PhasorSimulation=off  OutputType=Complex  PSBequivalent=0
  Current Measurement1 : powerlib/Measurements/Current Measurement  PhasorSimulation=off  OutputType=Complex  PSBequivalent=0
  Current Measurement2 : powerlib/Measurements/Current Measurement  PhasorSimulation=off  OutputType=Complex  PSBequivalent=0
  Mux : Mux  Inputs=3
  Mux1 : Mux  Inputs=3
  Voltage Measurement : powerlib/Measurements/Voltage Measurement  PhasorSimulation=off  OutputType=Complex  PSBequivalent=0
  Voltage Measurement1 : powerlib/Measurements/Voltage Measurement  PhasorSimulation=off  OutputType=Complex  PSBequivalent=0
  Voltage Measurement2 : powerlib/Measurements/Voltage Measurement  PhasorSimulation=off  OutputType=Complex  PSBequivalent=0
  A : PMIOPort  Port=1  Side=Left
  a : PMIOPort  Port=2  Side=Right
  B : PMIOPort  Port=3  Side=Left
  b : PMIOPort  Port=4  Side=Right
  C : PMIOPort  Port=5  Side=Left
  c : PMIOPort  Port=6  Side=Right
  N : PMIOPort  Port=7  Side=Left
  n : PMIOPort  Port=8  Side=Right
  V_abc : Outport
  I_abc : Outport  Port=2
  wires:
  Current Measurement1/1 -> Mux/2
  Mux1/1 -> V_abc/1
  Mux/1 -> I_abc/1
  Current Measurement/1 -> Mux/1
  Voltage Measurement/1 -> Mux1/1
  Current Measurement2/1 -> Mux/3
  Voltage Measurement1/1 -> Mux1/2
  Voltage Measurement2/1 -> Mux1/3
  connections:
  Current Measurement2/RConn1 -- c/RConn1
  Current Measurement/RConn1 -- a/RConn1
  Current Measurement1/RConn1 -- b/RConn1
  Voltage Measurement2/LConn1 -- C/RConn1 -- Current Measurement2/LConn1
  Voltage Measurement2/LConn2 -- Voltage Measurement1/LConn2 -- Voltage Measurement/LConn2 -- N/RConn1 -- n/RConn1
  Voltage Measurement1/LConn1 -- B/RConn1 -- Current Measurement1/LConn1
  Voltage Measurement/LConn1 -- A/RConn1 -- Current Measurement/LConn1

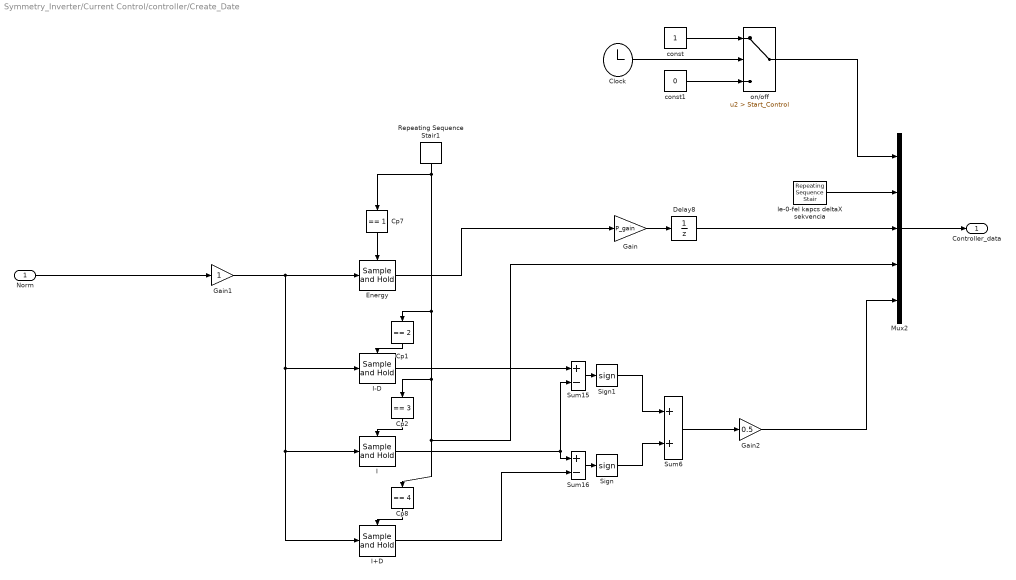
== system Symmetry_Inverter/Current Control/controller/Create_Date ==
  Norm : Inport
  Clock : Clock
      settings: Decimation=CLK
  Cp1 : simulink/Logic and Bit Operations/Compare To Constant  relop===  const=2  OutDataTypeStr=uint8  ZeroCross=off
  Cp2 : simulink/Logic and Bit Operations/Compare To Constant  relop===  const=3  OutDataTypeStr=uint8  ZeroCross=off
  Cp7 : simulink/Logic and Bit Operations/Compare To Constant  relop===  const=1  OutDataTypeStr=uint8  ZeroCross=off
  Cp8 : simulink/Logic and Bit Operations/Compare To Constant  relop===  const=4  OutDataTypeStr=uint8  ZeroCross=off
  Delay8 : UnitDelay  SampleTime=0.02
  Energy : dspsigops/Sample and Hold  trig=Rising edge  initCond=18  latchinput=off
  Gain : Gain  Gain=P_gain
  Gain1 : Gain
  Gain2 : Gain  Gain=0.5
  I : dspsigops/Sample and Hold  trig=Rising edge  initCond=0  latchinput=off
  I+D : dspsigops/Sample and Hold  trig=Rising edge  initCond=0  latchinput=off
  I-D : dspsigops/Sample and Hold  trig=Rising edge  initCond=0  latchinput=off
  Mux2 : Mux  Inputs=5
  Repeating Sequence Stair1 : simulink/Sources/Repeating Sequence Stair  OutValues=[1 2 3 4 5].'  tsamp=stair_sample  OutMin=[]  OutMax=[]  OutDataTypeStr=float('double')  OutputDataTypeScalingMode=Specify via dialog  OutDataType=float('double')  ConRadixGroup=Best Precision: Vector-wise  OutScaling=2^-12
  Sign : Signum
  Sign1 : Signum
  Sum15 : Sum  Inputs=+-
  Sum16 : Sum  Inputs=+-
  Sum6 : Sum
  const : Constant
  const1 : Constant  Value=0
  le-0-fel kapcs deltaX sekvencia : simulink/Sources/Repeating Sequence Stair  OutValues=[-1 0 1 0 0].'  tsamp=switch_sample  OutMin=[]  OutMax=[]  OutDataTypeStr=float('double')  OutputDataTypeScalingMode=Specify via dialog  OutDataType=float('double')  ConRadixGroup=Best Precision: Vector-wise  OutScaling=2^-12
  on/off : Switch  Criteria=u2 > Threshold  Threshold=Start_Control
  Controller_data : Outport
  wires:
  Cp1/1 -> I-D/Trigger
  Repeating Sequence Stair1/1 -> Cp7/1, Mux2/4, Cp8/1, Cp2/1, Cp1/1
  Cp7/1 -> Energy/Trigger
  Energy/1 -> Gain/1
  Cp2/1 -> I/Trigger
  Cp8/1 -> I+D/Trigger
  Gain1/1 -> I+D/1, I/1, I-D/1, Energy/1
  I-D/1 -> Sum15/1
  I/1 -> Sum15/2, Sum16/1
  I+D/1 -> Sum16/2
  Sum16/1 -> Sign/1
  Sum15/1 -> Sign1/1
  Gain/1 -> Delay8/1
  Sign/1 -> Sum6/2
  Sign1/1 -> Sum6/1
  le-0-fel kapcs deltaX sekvencia/1 -> Mux2/2
  Delay8/1 -> Mux2/3
  on/off/1 -> Mux2/1
  Mux2/1 -> Controller_data/1
  Norm/1 -> Gain1/1
  Sum6/1 -> Gain2/1
  const/1 -> on/off/1
  const1/1 -> on/off/3
  Clock/1 -> on/off/2
  Gain2/1 -> Mux2/5

== system Symmetry_Inverter/Current Control/controller/Phase_control_S ==
  Control : Inport
  Cp3 : simulink/Logic and Bit Operations/Compare To Constant  relop===  const=5  OutDataTypeStr=uint8  ZeroCross=off
  Delay : UnitDelay  SampleTime=0.001
  Delay4 : UnitDelay  SampleTime=0.02
  Demux2 : Demux  Outputs=5
  I Controller : dspsigops/Sample and Hold  trig=Rising edge  initCond=0  latchinput=off
  I3 Step : Constant  Value=step_size(5)
  "I3 init " : Constant  Value=initial_value(5)
  I3 test step : Constant  Value=test_step(5)
  Mask : simulink/Sources/Repeating Sequence Stair  OutValues=[0 0 0 0 1 0].'  tsamp=mask_sample  OutMin=[]  OutMax=[]  OutDataTypeStr=float('double')  OutputDataTypeScalingMode=Specify via dialog  OutDataType=float('double')  ConRadixGroup=Best Precision: Vector-wise  OutScaling=2^-12
  Product : Product  RndMeth=Zero
  Product12 : Product  RndMeth=Zero
  Product4 : Product  Inputs=4  RndMeth=Zero
  Product8 : Product  Inputs=4  RndMeth=Zero
  Saturation : Saturate  UpperLimit=phase_feedback_saturation  LowerLimit=-phase_feedback_saturation
  Sum : Sum  Inputs=|++
  Sum5 : Sum  Inputs=+++
  phase_S : Outport
  wires:
  Control/1 -> Demux2/1
  Product12/1 -> phase_S/1
  Product8/1 -> Sum/1
  Delay/1 -> Saturation/1
  "I3 init "/1 -> Sum5/2
  Delay4/1 -> Sum5/3
  Demux2/5 -> Product8/2
  Demux2/4 -> Product/2
  Demux2/3 -> Product4/3, Product8/1
  Demux2/2 -> Product4/2
  Demux2/1 -> Product12/1, Product8/4
  I3 Step/1 -> Product8/3
  Cp3/1 -> I Controller/Trigger
  Mask/1 -> Product/1, Product4/4
  Sum5/1 -> Product12/2
  I3 test step/1 -> Product4/1
  I Controller/1 -> Delay4/1, Delay/1
  Product4/1 -> Sum5/1
  Product/1 -> Cp3/1
  Sum/1 -> I Controller/1
  Saturation/1 -> Sum/2

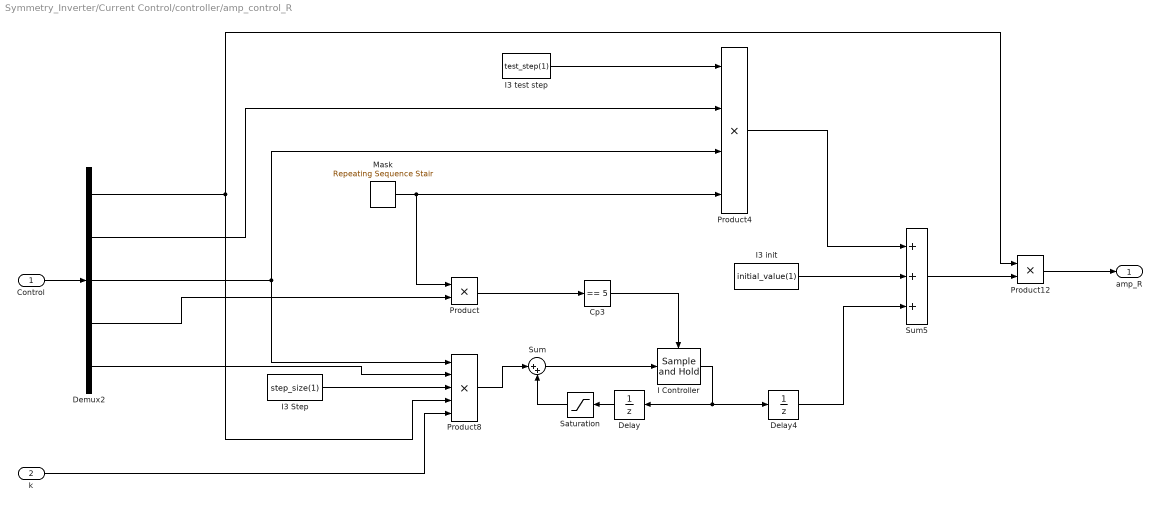
== system Symmetry_Inverter/Current Control/controller/amp_control_R ==
  Control : Inport
  k : Inport  Port=2
  Cp3 : simulink/Logic and Bit Operations/Compare To Constant  relop===  const=5  OutDataTypeStr=uint8  ZeroCross=off
  Delay : UnitDelay  SampleTime=0.001
  Delay4 : UnitDelay  SampleTime=0.02
  Demux2 : Demux  Outputs=5
  I Controller : dspsigops/Sample and Hold  trig=Rising edge  initCond=0  latchinput=off
  I3 Step : Constant  Value=step_size(1)
  "I3 init " : Constant  Value=initial_value(1)
  I3 test step : Constant  Value=test_step(1)
  Mask : simulink/Sources/Repeating Sequence Stair  OutValues=[1 0 0 0 0 0].'  tsamp=mask_sample  OutMin=[]  OutMax=[]  OutDataTypeStr=float('double')  OutputDataTypeScalingMode=Specify via dialog  OutDataType=float('double')  ConRadixGroup=Best Precision: Vector-wise  OutScaling=2^-12
  Product : Product  RndMeth=Zero
  Product12 : Product  RndMeth=Zero
  Product4 : Product  Inputs=4  RndMeth=Zero
  Product8 : Product  Inputs=5  RndMeth=Zero
  Saturation : Saturate  UpperLimit=amp_feedback_saturation  LowerLimit=-amp_feedback_saturation
  Sum : Sum  Inputs=|++
  Sum5 : Sum  Inputs=+++
  amp_R : Outport
  wires:
  Control/1 -> Demux2/1
  Product12/1 -> amp_R/1
  Product8/1 -> Sum/1
  Delay/1 -> Saturation/1
  "I3 init "/1 -> Sum5/2
  Delay4/1 -> Sum5/3
  Demux2/5 -> Product8/2
  Demux2/4 -> Product/2
  Demux2/3 -> Product4/3, Product8/1
  Demux2/2 -> Product4/2
  Demux2/1 -> Product12/1, Product8/4
  I3 Step/1 -> Product8/3
  Cp3/1 -> I Controller/Trigger
  Mask/1 -> Product/1, Product4/4
  Sum5/1 -> Product12/2
  I3 test step/1 -> Product4/1
  I Controller/1 -> Delay4/1, Delay/1
  Product4/1 -> Sum5/1
  Product/1 -> Cp3/1
  Sum/1 -> I Controller/1
  Saturation/1 -> Sum/2
  k/1 -> Product8/5

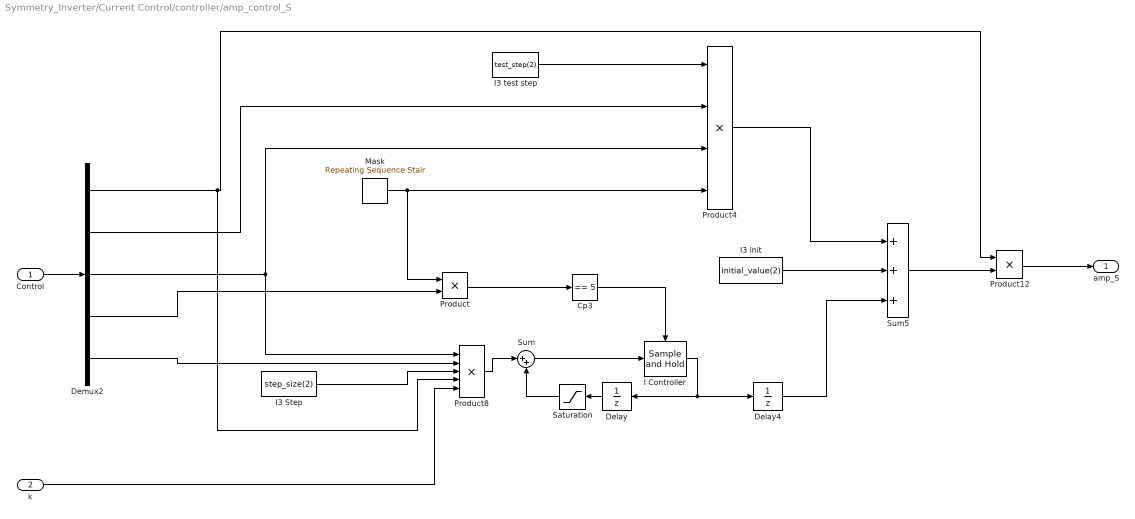
== system Symmetry_Inverter/Current Control/controller/amp_control_S ==
  Control : Inport
  k : Inport  Port=2
  Cp3 : simulink/Logic and Bit Operations/Compare To Constant  relop===  const=5  OutDataTypeStr=uint8  ZeroCross=off
  Delay : UnitDelay  SampleTime=0.001
  Delay4 : UnitDelay  SampleTime=0.02
  Demux2 : Demux  Outputs=5
  I Controller : dspsigops/Sample and Hold  trig=Rising edge  initCond=0  latchinput=off
  I3 Step : Constant  Value=step_size(2)
  "I3 init " : Constant  Value=initial_value(2)
  I3 test step : Constant  Value=test_step(2)
  Mask : simulink/Sources/Repeating Sequence Stair  OutValues=[0 1 0 0 0 0].'  tsamp=mask_sample  OutMin=[]  OutMax=[]  OutDataTypeStr=float('double')  OutputDataTypeScalingMode=Specify via dialog  OutDataType=float('double')  ConRadixGroup=Best Precision: Vector-wise  OutScaling=2^-12
  Product : Product  RndMeth=Zero
  Product12 : Product  RndMeth=Zero
  Product4 : Product  Inputs=4  RndMeth=Zero
  Product8 : Product  Inputs=5  RndMeth=Zero
  Saturation : Saturate  UpperLimit=amp_feedback_saturation  LowerLimit=-amp_feedback_saturation
  Sum : Sum  Inputs=|++
  Sum5 : Sum  Inputs=+++
  amp_S : Outport
  wires:
  Saturation/1 -> Sum/2
  Sum/1 -> I Controller/1
  Product/1 -> Cp3/1
  Product4/1 -> Sum5/1
  I Controller/1 -> Delay/1, Delay4/1
  I3 test step/1 -> Product4/1
  Sum5/1 -> Product12/2
  Mask/1 -> Product4/4, Product/1
  Cp3/1 -> I Controller/Trigger
  I3 Step/1 -> Product8/3
  Demux2/1 -> Product8/4, Product12/1
  Demux2/2 -> Product4/2
  Demux2/3 -> Product8/1, Product4/3
  Demux2/4 -> Product/2
  Demux2/5 -> Product8/2
  Delay4/1 -> Sum5/3
  "I3 init "/1 -> Sum5/2
  Delay/1 -> Saturation/1
  Product8/1 -> Sum/1
  Product12/1 -> amp_S/1
  Control/1 -> Demux2/1
  k/1 -> Product8/5

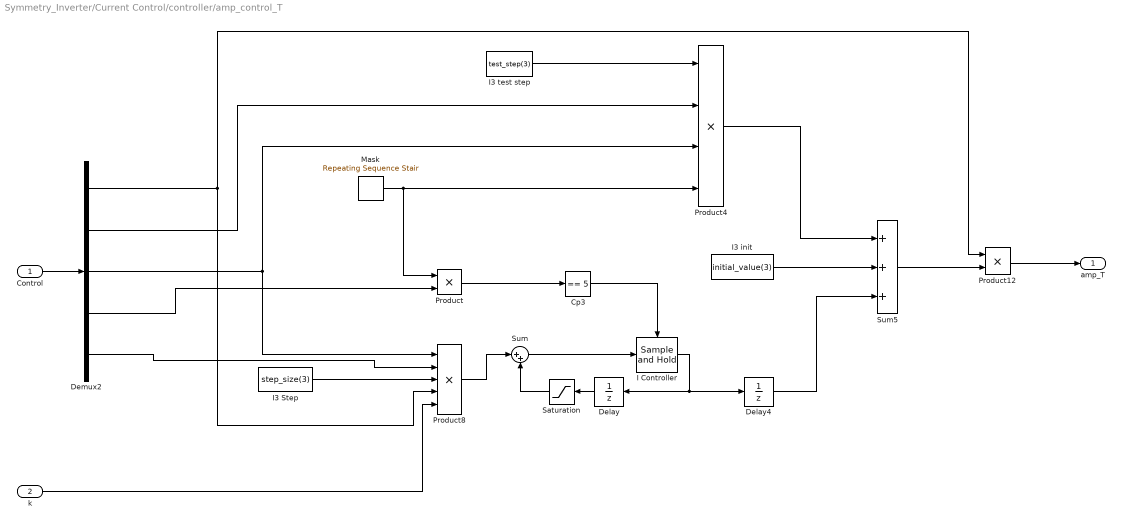
== system Symmetry_Inverter/Current Control/controller/amp_control_T ==
  Control : Inport
  k : Inport  Port=2
  Cp3 : simulink/Logic and Bit Operations/Compare To Constant  relop===  const=5  OutDataTypeStr=uint8  ZeroCross=off
  Delay : UnitDelay  SampleTime=0.001
  Delay4 : UnitDelay  SampleTime=0.02
  Demux2 : Demux  Outputs=5
  I Controller : dspsigops/Sample and Hold  trig=Rising edge  initCond=0  latchinput=off
  I3 Step : Constant  Value=step_size(3)
  "I3 init " : Constant  Value=initial_value(3)
  I3 test step : Constant  Value=test_step(3)
  Mask : simulink/Sources/Repeating Sequence Stair  OutValues=[0 0 1 0 0 0].'  tsamp=mask_sample  OutMin=[]  OutMax=[]  OutDataTypeStr=float('double')  OutputDataTypeScalingMode=Specify via dialog  OutDataType=float('double')  ConRadixGroup=Best Precision: Vector-wise  OutScaling=2^-12
  Product : Product  RndMeth=Zero
  Product12 : Product  RndMeth=Zero
  Product4 : Product  Inputs=4  RndMeth=Zero
  Product8 : Product  Inputs=5  RndMeth=Zero
  Saturation : Saturate  UpperLimit=amp_feedback_saturation  LowerLimit=-amp_feedback_saturation
  Sum : Sum  Inputs=|++
  Sum5 : Sum  Inputs=+++
  amp_T : Outport
  wires:
  Control/1 -> Demux2/1
  Product12/1 -> amp_T/1
  Product8/1 -> Sum/1
  Delay/1 -> Saturation/1
  "I3 init "/1 -> Sum5/2
  Delay4/1 -> Sum5/3
  Demux2/5 -> Product8/2
  Demux2/4 -> Product/2
  Demux2/3 -> Product4/3, Product8/1
  Demux2/2 -> Product4/2
  Demux2/1 -> Product12/1, Product8/4
  I3 Step/1 -> Product8/3
  Cp3/1 -> I Controller/Trigger
  Mask/1 -> Product/1, Product4/4
  Sum5/1 -> Product12/2
  I3 test step/1 -> Product4/1
  I Controller/1 -> Delay4/1, Delay/1
  Product4/1 -> Sum5/1
  Product/1 -> Cp3/1
  Sum/1 -> I Controller/1
  Saturation/1 -> Sum/2
  k/1 -> Product8/5

== system Symmetry_Inverter/Current Control/controller/phase_control_R ==
  Control : Inport
  Cp3 : simulink/Logic and Bit Operations/Compare To Constant  relop===  const=5  OutDataTypeStr=uint8  ZeroCross=off
  Delay : UnitDelay  SampleTime=0.001
  Delay4 : UnitDelay  SampleTime=0.02
  Demux2 : Demux  Outputs=5
  I Controller : dspsigops/Sample and Hold  trig=Rising edge  initCond=0  latchinput=off
  I3 Step : Constant  Value=step_size(4)
  "I3 init " : Constant  Value=initial_value(4)
  I3 test step : Constant  Value=test_step(4)
  Mask : simulink/Sources/Repeating Sequence Stair  OutValues=[0 0 0 1 0 0].'  tsamp=mask_sample  OutMin=[]  OutMax=[]  OutDataTypeStr=float('double')  OutputDataTypeScalingMode=Specify via dialog  OutDataType=float('double')  ConRadixGroup=Best Precision: Vector-wise  OutScaling=2^-12
  Product : Product  RndMeth=Zero
  Product12 : Product  RndMeth=Zero
  Product4 : Product  Inputs=4  RndMeth=Zero
  Product8 : Product  Inputs=4  RndMeth=Zero
  Saturation : Saturate  UpperLimit=phase_feedback_saturation  LowerLimit=-phase_feedback_saturation
  Sum : Sum  Inputs=|++
  Sum5 : Sum  Inputs=+++
  phase_R : Outport
  wires:
  Saturation/1 -> Sum/2
  Sum/1 -> I Controller/1
  Product/1 -> Cp3/1
  Product4/1 -> Sum5/1
  I Controller/1 -> Delay/1, Delay4/1
  I3 test step/1 -> Product4/1
  Sum5/1 -> Product12/2
  Mask/1 -> Product4/4, Product/1
  Cp3/1 -> I Controller/Trigger
  I3 Step/1 -> Product8/3
  Demux2/1 -> Product12/1, Product8/4
  Demux2/2 -> Product4/2
  Demux2/3 -> Product8/1, Product4/3
  Demux2/4 -> Product/2
  Demux2/5 -> Product8/2
  Delay4/1 -> Sum5/3
  "I3 init "/1 -> Sum5/2
  Delay/1 -> Saturation/1
  Product8/1 -> Sum/1
  Product12/1 -> phase_R/1
  Control/1 -> Demux2/1

== system Symmetry_Inverter/Current Control/controller/phase_control_T ==
  Control : Inport
  Cp3 : simulink/Logic and Bit Operations/Compare To Constant  relop===  const=5  OutDataTypeStr=uint8  ZeroCross=off
  Delay : UnitDelay  SampleTime=0.001
  Delay4 : UnitDelay  SampleTime=0.02
  Demux2 : Demux  Outputs=5
  I Controller : dspsigops/Sample and Hold  trig=Rising edge  initCond=0  latchinput=off
  I3 Step : Constant  Value=step_size(6)
  "I3 init " : Constant  Value=initial_value(6)
  I3 test step : Constant  Value=test_step(6)
  Mask : simulink/Sources/Repeating Sequence Stair  OutValues=[0 0 0 0 0 1].'  tsamp=mask_sample  OutMin=[]  OutMax=[]  OutDataTypeStr=float('double')  OutputDataTypeScalingMode=Specify via dialog  OutDataType=float('double')  ConRadixGroup=Best Precision: Vector-wise  OutScaling=2^-12
  Product : Product  RndMeth=Zero
  Product12 : Product  RndMeth=Zero
  Product4 : Product  Inputs=4  RndMeth=Zero
  Product8 : Product  Inputs=4  RndMeth=Zero
  Saturation : Saturate  UpperLimit=phase_feedback_saturation  LowerLimit=-phase_feedback_saturation
  Sum : Sum  Inputs=|++
  Sum5 : Sum  Inputs=+++
  phase_S : Outport
  wires:
  Saturation/1 -> Sum/2
  Sum/1 -> I Controller/1
  Product/1 -> Cp3/1
  Product4/1 -> Sum5/1
  I Controller/1 -> Delay/1, Delay4/1
  I3 test step/1 -> Product4/1
  Sum5/1 -> Product12/2
  Mask/1 -> Product4/4, Product/1
  Cp3/1 -> I Controller/Trigger
  I3 Step/1 -> Product8/3
  Demux2/1 -> Product12/1, Product8/4
  Demux2/2 -> Product4/2
  Demux2/3 -> Product8/1, Product4/3
  Demux2/4 -> Product/2
  Demux2/5 -> Product8/2
  Delay4/1 -> Sum5/3
  "I3 init "/1 -> Sum5/2
  Delay/1 -> Saturation/1
  Product8/1 -> Sum/1
  Product12/1 -> phase_S/1
  Control/1 -> Demux2/1
